simulink model "projemodel3"  (R2019a)
settings: Solver=VariableStepAuto  StartTime=0.0  StopTime=200  RelTol=1e-3
values from neighbouring files (symbols this model uses):
  Am = [ 1 1 1/2;0 1 1;0 0 1]    [Untitled.m]    (also in projematlabcod.m)
  Bm = [0 ; 0; 1/80]    [Untitled.m]    (also in projematlabcod.m)
  Cm = [1 0 0]    [Untitled.m]    (also in projematlabcod.m)
  Dm = 1    [Untitled.m]    (also in projematlabcod.m)
  initilizecondition = [0.00001 0 0 ]    [Untitled.m]
  K = lqr(systeml,Q,R)    [Untitled.m]
undefined symbols (not defined in the file or in its folder): Continuous, Time
libraries: ctrlSharedLib x2
settings Model: Creator=tr531  LastModifiedBy=tr531

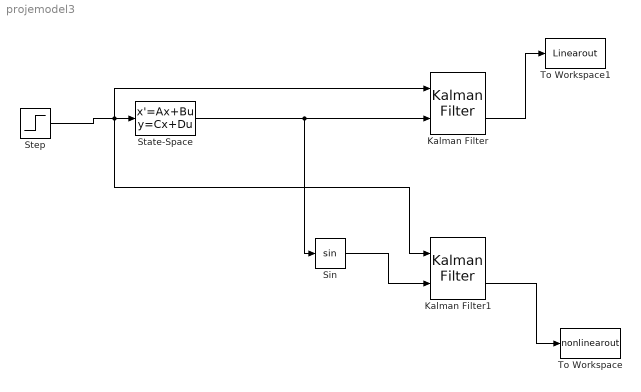
== system projemodel3 ==
  Kalman Filter : ctrlSharedLib/Kalman Filter  TimeDomain=Continuous-Time  UseCurrentEstimator=on  ModelSource=Individual A, B, C, D matrices  ModelSourceVariable=ss(0.95,1,1,0,1)  A=[1 1 0.5;0 1 1;0 0 1]  B=[0 ;0 ;0.125]  C=[1 0 0]  D=1  NumberOfStates=1  NumberOfInputs=1  NumberOfOutputs=1  InitialEstimateSource=Dialog  X0=0  P0=10  UseK=off  UseGH=off  NumberOfProcessNoiseInputs=1  G=1  TimeInvariantG=on  H=0  TimeInvariantH=on  Q=1  TimeInvariantQ=on  R=1  TimeInvariantR=on  N=0  TimeInvariantN=on  AddInputPort=on  AddEnablePort=off  OutputEstimatedY=on  OutputP=off  Ts=-1
      settings: SourceProductBaseCode=CT
  Kalman Filter1 : ctrlSharedLib/Kalman Filter  TimeDomain=Continuous-Time  UseCurrentEstimator=on  ModelSource=Individual A, B, C, D matrices  ModelSourceVariable=ss(0.95,1,1,0,1)  A=[1 1 0.5;0 1 1;0 0 1]  B=[0 ;0 ;0.125]  C=[1 0 0]  D=1  NumberOfStates=1  NumberOfInputs=1  NumberOfOutputs=1  InitialEstimateSource=Dialog  X0=0  P0=10  UseK=off  UseGH=off  NumberOfProcessNoiseInputs=1  G=1  TimeInvariantG=on  H=0  TimeInvariantH=on  Q=1  TimeInvariantQ=on  R=1  TimeInvariantR=on  N=0  TimeInvariantN=on  AddInputPort=on  AddEnablePort=off  OutputEstimatedY=on  OutputP=off  Ts=-1
      settings: SourceProductBaseCode=CT
  Sin : Trigonometry
  State-Space : StateSpace  A=Am-Bm*K  B=zeros(size(Bm))  C=Cm-Dm*K  D=zeros(size(Dm))  InitialCondition=initilizecondition
  Step : Step  Time=0  After=0  SampleTime=0
  To Workspace : ToWorkspace  VariableName=nonlinearout  SaveFormat=Timeseries  SampleTime=-1
  To Workspace1 : ToWorkspace  VariableName=Linearout  SaveFormat=Timeseries  SampleTime=-1
  wires:
  State-Space/1 -> Sin/1, Kalman Filter/2
  Step/1 -> Kalman Filter1/1, Kalman Filter/1, State-Space/1
  Kalman Filter/2 -> To Workspace1/1
  Sin/1 -> Kalman Filter1/2
  Kalman Filter1/2 -> To Workspace/1
